simulink model "Planta_completa_controle_velocidade"  (R2023b)
settings: Solver=VariableStepAuto  StartTime=0.0  StopTime=10.0  RelTol=1e-3
values from neighbouring files (symbols this model uses):
  Cmn = Pmec / Wn    (= 479.991198073)    [minimos_quadrados_matlab.m]    (also in parametros_do_motor.m; realimentacao_de_estados.m)
  J = 0.56    [minimos_quadrados_matlab.m]    (also in parametros_do_motor.m; realimentacao_de_estados.m)
  Kf = (Vn - Ian * Ra) / Wn    (= 1.91586963478)    [minimos_quadrados_matlab.m]    (also in parametros_do_motor.m; realimentacao_de_estados.m)
  La = 1.4 * 10^-3    (= 0.0014)    [minimos_quadrados_matlab.m]    (also in parametros_do_motor.m; realimentacao_de_estados.m)
  T = Te/10    (= 0.00175)    [minimos_quadrados_matlab.m]    (also in parametros_do_motor.m; projeto_controlador_corrente_velocidade.m; projeto_controlador_velocidade.m; projeto_controlador_w.m)
  Te = La / Ra    (= 0.0175)    [minimos_quadrados_matlab.m]    (also in parametros_do_motor.m; realimentacao_de_estados.m)
  Tm = J / B    (= 6.02801217209)    [minimos_quadrados_matlab.m]    (also in parametros_do_motor.m; realimentacao_de_estados.m)
  Vn = 400    [minimos_quadrados_matlab.m]    (also in parametros_do_motor.m; realimentacao_de_estados.m)
  Wn = 1890 * 3.141592 / 30    (= 197.920296)    [minimos_quadrados_matlab.m]    (also in parametros_do_motor.m; realimentacao_de_estados.m)
libraries: simulink x3
settings Model: Creator=lpds  LastModifiedBy=lpds

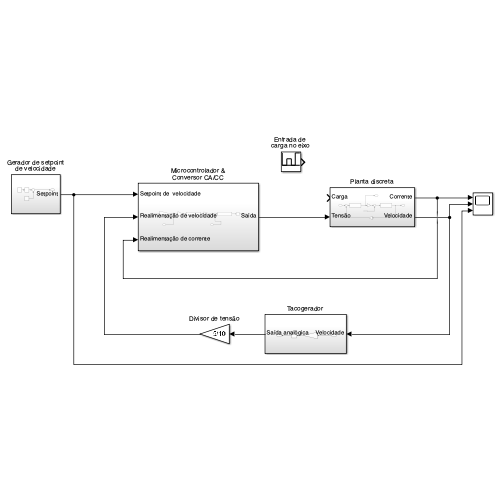
[thumbnail: Simulink's stored preview of the top-level diagram]
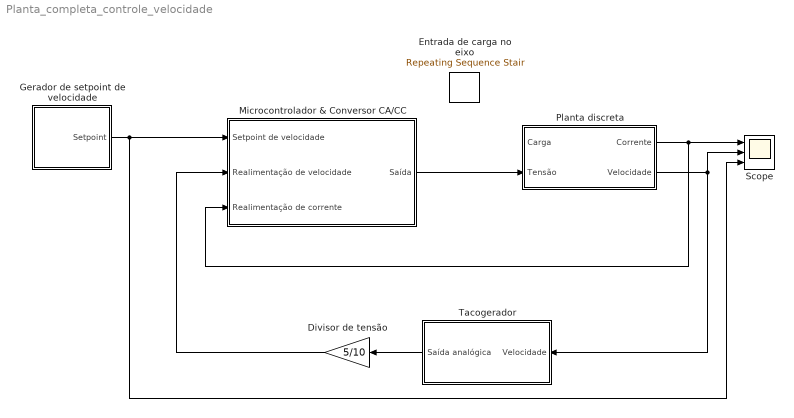
== system Planta_completa_controle_velocidade ==
  Divisor de tensão : Gain  Gain=5/10
  Entrada de carga no eixo : simulink/Sources/Repeating Sequence Stair  OutValues=[0 Cmn 0 2*Cmn]  tsamp=858 * 0.00175  OutMin=[]  OutMax=[]  OutDataTypeStr=double  OutputDataTypeScalingMode=double  OutDataType=fixdt(0,8)  ConRadixGroup=Best Precision: Vector-wise  OutScaling=2^-12
  Gerador de setpoint de velocidade : Subsystem
  Microcontrolador & Conversor CA/CC : Subsystem
  Planta discreta : Subsystem
  Scope : Scope  NumInputPorts=3
  Tacogerador : Subsystem
  wires:
  Tacogerador/1(Saída analógica) -> Divisor de tensão/1
  Gerador de setpoint de velocidade/1(Setpoint) -> Scope/3, Microcontrolador & Conversor CA/CC/1(Setpoint de velocidade)
  Divisor de tensão/1 -> Microcontrolador & Conversor CA/CC/2(Realimentação de velocidade)
  Planta discreta/2(Velocidade) -> Scope/2, Tacogerador/1(Velocidade)
  Planta discreta/1(Corrente) -> Microcontrolador & Conversor CA/CC/3(Realimentação de corrente), Scope/1
  Microcontrolador & Conversor CA/CC/1(Saída) -> Planta discreta/2(Tensão)

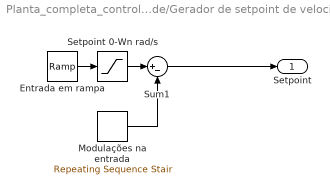
== system Planta_completa_controle_velocidade/Gerador de setpoint de velocidade ==
  Entrada em rampa : simulink/Sources/Ramp  slope=Wn*2  start=0  InitialOutput=0
  Modulações na entrada : simulink/Sources/Repeating Sequence Stair  OutValues=[0 50 -50].'  tsamp=1143 * 0.00175  OutMin=[]  OutMax=[]  OutDataTypeStr=double  OutputDataTypeScalingMode=double  OutDataType=fixdt(0,8)  ConRadixGroup=Best Precision: Vector-wise  OutScaling=2^-12
  Setpoint 0-Wn rad/s : Saturate  UpperLimit=Wn
  Sum1 : Sum  Inputs=|+-
  Setpoint : Outport
  wires:
  Sum1/1 -> Setpoint/1
  Entrada em rampa/1 -> Setpoint 0-Wn rad/s/1
  Setpoint 0-Wn rad/s/1 -> Sum1/1
  Modulações na entrada/1 -> Sum1/2

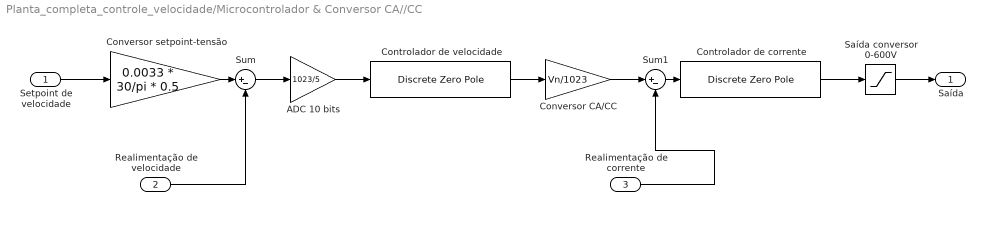
== system Planta_completa_controle_velocidade/Microcontrolador & Conversor CA//CC ==
  Setpoint de velocidade : Inport
  Realimentação de velocidade : Inport  Port=2
  Realimentação de corrente : Inport  Port=3
  "ADC 10 bits " : Gain  Gain=1023/5
  Controlador de velocidade : DiscreteZeroPole  Zeros=[0.9]  Poles=[1]  Gain=0.1  SampleTime=T
  Controlador de corrente : DiscreteZeroPole  Zeros=[0.9]  Poles=[1]  Gain=0.1  SampleTime=T
  Conversor setpoint-tensão : Gain  Gain=0.0033 * 30/pi * 0.5
  Conversor CA/CC : Gain  Gain=Vn/1023
  Saída conversor 0-600V : Saturate  UpperLimit=600  LowerLimit=0
  Sum : Sum  Inputs=|+-
  Sum1 : Sum  Inputs=|+-
  Saída : Outport
  wires:
  Realimentação de velocidade/1 -> Sum/2
  Sum/1 -> "ADC 10 bits "/1
  "ADC 10 bits "/1 -> Controlador de velocidade/1
  Conversor setpoint-tensão/1 -> Sum/1
  Saída conversor 0-600V/1 -> Saída/1
  Setpoint de velocidade/1 -> Conversor setpoint-tensão/1
  Controlador de velocidade/1 -> Conversor CA/CC/1
  Conversor CA/CC/1 -> Sum1/1
  Sum1/1 -> Controlador de corrente/1
  Controlador de corrente/1 -> Saída conversor 0-600V/1
  Realimentação de corrente/1 -> Sum1/2

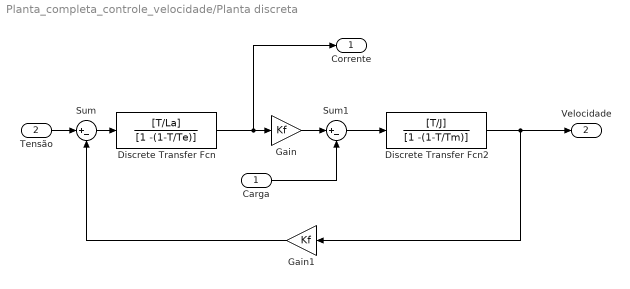
== system Planta_completa_controle_velocidade/Planta discreta ==
  Carga : Inport
  Tensão : Inport  Port=2
  Discrete Transfer Fcn : DiscreteTransferFcn  Numerator=[T/La]  Denominator=[1 -(1-T/Te)]
  Discrete Transfer Fcn2 : DiscreteTransferFcn  Numerator=[T/J]  Denominator=[1 -(1-T/Tm)]
  Gain : Gain  Gain=Kf
  Gain1 : Gain  Gain=Kf
  Sum : Sum  Inputs=|+-
  Sum1 : Sum  Inputs=|+-
  Corrente : Outport
  Velocidade : Outport  Port=2
  wires:
  Gain/1 -> Sum1/1
  Gain1/1 -> Sum/2
  Sum/1 -> Discrete Transfer Fcn/1
  Carga/1 -> Sum1/2
  Discrete Transfer Fcn2/1 -> Velocidade/1, Gain1/1
  Sum1/1 -> Discrete Transfer Fcn2/1
  Tensão/1 -> Sum/1
  Discrete Transfer Fcn/1 -> Corrente/1, Gain/1

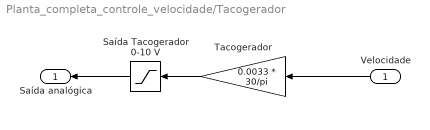
== system Planta_completa_controle_velocidade/Tacogerador ==
  Velocidade : Inport
  Saída Tacogerador 0-10 V : Saturate  UpperLimit=10  LowerLimit=0
  Tacogerador : Gain  Gain=0.0033 * 30/pi
  Saída analógica : Outport
  wires:
  Velocidade/1 -> Tacogerador/1
  Saída Tacogerador 0-10 V/1 -> Saída analógica/1
  Tacogerador/1 -> Saída Tacogerador 0-10 V/1
